simulink model "Clutchless_P2_Parallel_ETE"  (R2017b)
settings: Solver=FixedStepAuto  StartTime=0.0  StopTime=length(Speed)  FixedStep=0.01  MaxStep=0.01  RelTol=1e-3  EnableMultiTasking=on
PostLoadFcn:
  | , if any(exist('dsrtsu_mdlpostloadfcn', 'file') == [2, 3, 6]), try dsrtsu_mdlpostloadfcn('Execute', bdroot); catch fprintf('Error in PostLoadFcn (dsrtsu_mdlpostloadfcn) for model "%s":\n %s\n', bdroot, lasterr); end, end,
undefined symbols (not defined in the file): ABSEnable, Actuators, air, APP1_OOR, APP2_OOR, APP_Mismatch, Brk_Flt, cal, ClutchEngag, Clutchless_HSC_ETE, CS_On_Control, Driver, eng, Engine, EngOverTemp, ENGTRQ_MSMCH_Degraded_CP, ENGTRQ_MSMCH_ErrCritical_CP, ENGTRQ_MSMCH_LimpHome_CP, EngTrqMismatch, env, ess, ESSOverTemp, gb, KeyPos_Flt, KeyPosition, lib_Actuators, lib_Clutchless_HSC_ETE, lib_Driver, lib_EMachine_2017a, lib_Sensors_2017a, LossCAN, Machine, max_vehicle_rad_air_flow, MCUOverTemp, mot, MotDirMismatch, MotOverTemp, MotTrqMismatch, mph2ms, PRNDL_Flt, RegenBrkDisable, RegenFault, Sensors, ShiftLeverPosition, Speed, SW_CS_ON, SW_Engine_ON, t_amb, time, tloop
libraries: simulink x97, Pneumatic_lib x11, nesl_utility x9, EC2_libraries x7, powerlib_meascontrol x2, CalculationGallon x1, lib_Chassis x1, lib_DCDC x1, lib_Differential x1, lib_HVESS x1, fl_lib x1, lib_OBC x1
(part 5 of 9)

== system Clutchless_P2_Parallel_ETE/Clutchless_HSC_ETE/HSC/Camaro Fault Detection/Input Conversions/ECM_Conversions ==
  note: ECM: Input Conversions and Override Switches
      | (Engine and ECM)
  In1 : Inport
  Bus Creator : BusCreator  Inputs=6
  Bus Selector : BusSelector  OutputSignals=from_CAN.fromEBCAN.from_ECM.PlatEngSpdCmdStARC,from_CAN.fromEBCAN.from_ECM.EngSpd,from_CAN.fromEBCAN.from_ECM.EngCltTmp,from_CAN.fromEBCAN.from_ECM.EngRunAtv,from_CAN.fromEBCAN.from_ECM.EngActStdyStTorq
  Conversion  ECMTrqCmd_Nm : DataTypeConversion  OutDataTypeStr=double
  Conversion  EngActStdyStTorq_Nm : DataTypeConversion  OutDataTypeStr=double
  Conversion  EngRunAtv : DataTypeConversion  OutDataTypeStr=boolean
  Conversion  Engine_Speed_rpm : DataTypeConversion  OutDataTypeStr=double
  Conversion  Engine_Temp[DegC] : DataTypeConversion  OutDataTypeStr=double
  Conversion  rollingAliveCnt : DataTypeConversion  OutDataTypeStr=int8
  Memory : Memory
  Override  ECMTrqCmd_Nm : Subsystem
  Override  ECMrollingAliveCnt : Subsystem
  Override  EngActStdyStTorq_Nm : Subsystem
  Override  EngRunAtv : Subsystem
  Override  EngineSpeed_rpm : Subsystem
  Override  Engine_Temp[DegC] : Subsystem
  Out1 : Outport
  wires:
  In1/1 -> Bus Selector/1
  Conversion  rollingAliveCnt/1 -> Override  ECMrollingAliveCnt/1(In1)
  Override  ECMrollingAliveCnt/1(Out1) -> Bus Creator/1  "ECMrollingAliveCnt [123]"
  Bus Creator/1 -> Out1/1  "ECM_Conv"
  Override  ECMTrqCmd_Nm/1(Out1) -> Bus Creator/2  "ECMTrqCmd_Nm"
  Conversion  ECMTrqCmd_Nm/1 -> Override  ECMTrqCmd_Nm/1(In1)
  Bus Selector/2 -> Conversion  Engine_Speed_rpm/1  "<EngSpd>"
  Conversion  Engine_Speed_rpm/1 -> Override  EngineSpeed_rpm/1(In1)
  Override  EngineSpeed_rpm/1(Out1) -> Bus Creator/3  "EngineSpeed_rpm"
  Bus Selector/3 -> Conversion  Engine_Temp[DegC]/1  "<EngCltTmp>"
  Bus Selector/4 -> Conversion  EngRunAtv/1  "<EngRunAtv>"
  Bus Selector/5 -> Conversion  EngActStdyStTorq_Nm/1  "<EngActStdyStTorq>"
  Conversion  Engine_Temp[DegC]/1 -> Override  Engine_Temp[DegC]/1(In1)
  Conversion  EngRunAtv/1 -> Override  EngRunAtv/1(In1)
  Conversion  EngActStdyStTorq_Nm/1 -> Override  EngActStdyStTorq_Nm/1(In1)
  Override  Engine_Temp[DegC]/1(Out1) -> Bus Creator/4  "Engine_Temp[DegC]"
  Override  EngRunAtv/1(Out1) -> Bus Creator/5  "EngRunAtv"
  Override  EngActStdyStTorq_Nm/1(Out1) -> Bus Creator/6  "EngActStdyStTorq_Nm"
  Bus Selector/1 -> Conversion  rollingAliveCnt/1  "<PlatEngSpdCmdStARC>"
  [AxlEngTrqCmd] -> Memory/1
  Memory/1 -> Conversion  ECMTrqCmd_Nm/1

== system Clutchless_P2_Parallel_ETE/Clutchless_HSC_ETE/HSC/Camaro Fault Detection/Input Conversions/TCM_Conversions ==
  note: TCM: Input Conversions and Override Switches
      | (Transmission Control Module)
  In1 : Inport
  Bus Creator : BusCreator  Inputs=4
  Bus Selector : BusSelector  OutputSignals=from_CAN.fromVEH_CAN.from_TCM.TrnsShftLvrPos,from_CAN.fromVEH_CAN.from_TCM.TransEstGear,from_CAN.fromVEH_CAN.from_TCM.TrnsTrqCnvCltCmndMd
  Conversion  LockupCmd : DataTypeConversion  OutDataTypeStr=boolean
  Conversion  LvrPosTrnsShft : DataTypeConversion  OutDataTypeStr=int8
  Conversion  TransEstGear : DataTypeConversion  OutDataTypeStr=int8
  Conversion  rollingAliveCnt : DataTypeConversion  OutDataTypeStr=int8
  Override  LockupCmd : Subsystem
  "Override  LvrPosTrnsShft " : Subsystem
  Override  TransEstGear : Subsystem
  Override  rollingAliveCnt [123] : Subsystem
  TCM_RollinAliveCounter : Subsystem
  Out1 : Outport
  wires:
  Override  LockupCmd/1(Out1) -> Bus Creator/4  "LockupCmd_0_1"
  Conversion  LockupCmd/1 -> Override  LockupCmd/1(In1)
  Bus Selector/3 -> Conversion  LockupCmd/1  "<TrnsTrqCnvCltCmndMd>"
  Override  TransEstGear/1(Out1) -> Bus Creator/3  "TransEstGear"
  Conversion  TransEstGear/1 -> Override  TransEstGear/1(In1)
  Bus Selector/2 -> Conversion  TransEstGear/1  "<TransEstGear>"
  Conversion  LvrPosTrnsShft/1 -> "Override  LvrPosTrnsShft "/1(In1)
  "Override  LvrPosTrnsShft "/1(Out1) -> Bus Creator/2  "LvrPosTrnsShft"
  Bus Selector/1 -> Conversion  LvrPosTrnsShft/1  "<TrnsShftLvrPos>"
  Bus Creator/1 -> Out1/1  "TCM_Conv"
  Override  rollingAliveCnt [123]/1(Out1) -> Bus Creator/1  "TCMrollingAliveCnt [123]"
  Conversion  rollingAliveCnt/1 -> Override  rollingAliveCnt [123]/1(In1)
  In1/1 -> Bus Selector/1
  TCM_RollinAliveCounter/1(Out1) -> Conversion  rollingAliveCnt/1

== system Clutchless_P2_Parallel_ETE/Clutchless_HSC_ETE/HSC/Camaro Fault Detection/Signal Diagnostic/Driver Signal Diagnostic ==
  note: Driver Controls : Signal Diagnostic
  Sensors1 : Inport
  APP_Crosscheck : Subsystem
  AccPedalValidity : Stateflow chart  TreatAsAtomicUnit=on
  AccPedalValidity1 : Stateflow chart  TreatAsAtomicUnit=on
  BPP_faild_ovrd : Constant  Value=0  OutDataTypeStr=boolean
  BrakeFailureDetection : Subsystem
  Bus Creator : BusCreator  Inputs=7
  Bus Selector : BusSelector  OutputSignals=DriverControls_Conv.APP1 [%],DriverControls_Conv.APP2[%],DriverControls_Conv.BPP [%],DriverControls_Conv.V [mph],DriverControls_Conv.keyPos [0_3],DriverControls_Conv.PRNDL
  ClearAPP1fault : Constant  Value=0
  ClearAPP2fault : Constant  Value=0
  Constant2 : Constant  Value=0
  Constant3 : Constant  OutDataTypeStr=boolean
  Conversion  APP1 (%)1 : DataTypeConversion  OutDataTypeStr=boolean
  Conversion  APP1 (%)2 : DataTypeConversion
  Conversion  APP1 (%)3 : DataTypeConversion
  Drv_APP1_valid_ovrd : Constant  Value=0  OutDataTypeStr=boolean
  Drv_APP2_valid_ovrd : Constant  Value=0  OutDataTypeStr=boolean
  Interval Test : simulink/Logic and Bit Operations/Interval Test  IntervalClosedRight=on  uplimit=100  IntervalClosedLeft=on  lowlimit=0  OutDataTypeStr=boolean
  Interval Test1 : simulink/Logic and Bit Operations/Interval Test  IntervalClosedRight=on  uplimit=3  IntervalClosedLeft=on  lowlimit=0  OutDataTypeStr=boolean
  Interval Test2 : simulink/Logic and Bit Operations/Interval Test  IntervalClosedRight=on  uplimit=4  IntervalClosedLeft=on  lowlimit=0  OutDataTypeStr=boolean
  Latch : Subsystem
  Latch1 : Subsystem
  Logical Operator1 : Logic  AllPortsSameDT=off  OutDataTypeStr=boolean
  Logical Operator5 : Logic  Operator=OR  AllPortsSameDT=off  OutDataTypeStr=boolean
  Logical Operator6 : Logic  Operator=OR  AllPortsSameDT=off  OutDataTypeStr=boolean
  Pulse Generator : DiscretePulseGenerator  PulseType=Time based  Period=0.1  PulseWidth=10
  Scope : Scope
  Driver_SigDiag : Outport
  wires:
  Sensors1/1 -> Bus Selector/1
  Bus Selector/1 -> AccPedalValidity/2(signalValue), APP_Crosscheck/1(In1)  "<APP1 [%]>"
  Bus Selector/2 -> AccPedalValidity1/2(signalValue), APP_Crosscheck/2(In2)  "<APP2[%]>"
  ClearAPP1fault/1 -> AccPedalValidity/1(clearFaults)
  ClearAPP2fault/1 -> AccPedalValidity1/1(clearFaults)
  Bus Selector/3 -> Interval Test/1, BrakeFailureDetection/1(BPP)  "<BPP [%]>"
  Bus Selector/5 -> Interval Test1/1  "<keyPos [0_3]>"
  Logical Operator6/1 -> Bus Creator/1  "Drv_APP1_[%]_SigValid"
  Interval Test/1 -> Bus Creator/4  "Drv_BPP_[%]_SigValid"
  Logical Operator5/1 -> Bus Creator/2  "Drv_APP2_[%]_SigValid"
  Bus Creator/1 -> Driver_SigDiag/1  "Driver_SignalDiag"
  Bus Selector/6 -> Interval Test2/1  "<PRNDL>"
  Constant3/1 -> Latch/2(In2)
  APP_Crosscheck/1(Out1) -> Latch/1(In1)  "Drv_APP_Agree"
  Bus Selector/4 -> BrakeFailureDetection/2(VehSpeed)  "<V [mph]>"
  Constant2/1 -> Conversion  APP1 (%)1/1
  Conversion  APP1 (%)1/1 -> Latch1/2(In2)
  BrakeFailureDetection/1(DecelFail) -> Latch1/1(In1)  "Brake_Failed"
  Interval Test2/1 -> Bus Creator/7  "Drv_PRNDL_SigValid"
  Drv_APP2_valid_ovrd/1 -> Logical Operator5/1
  AccPedalValidity1/1(signalValid) -> Logical Operator5/2  "Drv_APP2_[%]_SigValid"
  Drv_APP1_valid_ovrd/1 -> Logical Operator6/1
  AccPedalValidity/1(signalValid) -> Logical Operator6/2  "Drv_APP1_[%]_SigValid"
  Conversion  APP1 (%)3/1 -> Bus Creator/3  "Drv_APP_Agree"
  Conversion  APP1 (%)2/1 -> Bus Creator/5  "Brake_Failed"
  Interval Test1/1 -> Bus Creator/6  "Drv_KeyPos_[0 3]_SigValid"
  Latch/1(Drv_APP_Agree) -> Conversion  APP1 (%)3/1  "Drv_APP_Agree"
  Logical Operator1/1 -> Conversion  APP1 (%)2/1  "Brake_Failed"
  Latch1/1(Out1) -> Logical Operator1/2  "Brake_Failed"
  BPP_faild_ovrd/1 -> Logical Operator1/1
  Pulse Generator/1 -> BrakeFailureDetection/Trigger, Scope/1

== system Clutchless_P2_Parallel_ETE/Clutchless_HSC_ETE/HSC/Camaro Fault Detection/Signal Diagnostic/ESS Signal Diagnostic ==
  note: max charge current: 180A
      | Max discharge current: 315A;
  note: Error: contactors welded,Contactors don't close when commanded
  note: Temperature Range check :
      | 0 = below normal operation (<-28)
      | 1 = low range (<0 - >-28)
      | 2 = normal range (0 -30 C)
      | 3= high range (>30)
      | 4= above max value allowed (>55)
  note: SOC Range check definition :
      | 0 = below normal operation (<0.15)
      | 1 = low range ([0.15 0.30])
      | 2 = normal range (0.3)
      | 3= SOC high/full (>0.95)
  note: 1) Rolling alive detection : is the component on and transmitting?
      | 2) Probably move the voltage check to component diagnostic (no signal from Bosch to check the contactors status)
      | 3) Is  the T signal within an acceptable range?
  note: BMS : Signal Diagnostic
  Sensors1 : Inport
  Bus Creator : BusCreator  Inputs=14
  Bus Selector : BusSelector  OutputSignals=BMS_Conv.BMSrollingAliveCnt [123],BMS_Conv.hvBattVolt_V,BMS_Conv.hvBusVolt_V,BMS_Conv.Fehler_HS_offen,BMS_Conv.MO_BMS_Sollmodus [0-5],BMS_Conv.Fehler_HS_verschweisst,BMS_Conv.essTemp_C,BMS_Conv.essSOC_0_1,BMS_Conv.essCur_A,BMS_Conv.BMS_gdf
  Contactors status check : Subsystem
  ESS SOC Validity Check : Subsystem
  ESS Temp Validity Check : Subsystem
  Interval Test : simulink/Logic and Bit Operations/Interval Test  IntervalClosedRight=on  uplimit=180  IntervalClosedLeft=on  lowlimit=-315  OutDataTypeStr=boolean
  Interval Test1 : simulink/Logic and Bit Operations/Interval Test  IntervalClosedRight=on  uplimit=7  IntervalClosedLeft=on  lowlimit=0  OutDataTypeStr=boolean
  Interval Test2 : simulink/Logic and Bit Operations/Interval Test  IntervalClosedRight=on  uplimit=430  IntervalClosedLeft=on  lowlimit=291  OutDataTypeStr=boolean
  Logical Operator : Logic  Operator=OR  AllPortsSameDT=off  OutDataTypeStr=boolean
  Max charging voltage fault detect : Subsystem
  Override_ BMS_RACvalid1 : Constant  Value=0
  Rolling Alive Counter Detection : Subsystem
  Validity Check : Subsystem
  ESS_SigDiag : Outport
  wires:
  Sensors1/1 -> Bus Selector/1
  Bus Selector/1 -> Rolling Alive Counter Detection/1(In1)  "<BMSrollingAliveCnt [123]>"
  Logical Operator/1 -> Bus Creator/1  "BMS_RollingAliveActive_SigValid"
  Bus Selector/2 -> Interval Test2/1, [BattVolt]  "<hvBattVolt_V>"
  Bus Creator/1 -> ESS_SigDiag/1  "ESS_SignalDiag"
  Bus Selector/9 -> Interval Test/1  "<essCur_A>"
  Interval Test/1 -> Bus Creator/12  "essCur_A_SigValid"
  Bus Selector/10 -> Bus Creator/14, Validity Check/1(In1)  "<BMS_gdf>"
  Validity Check/1(Out1) -> Bus Creator/13  "BMSgdf_SigValid"
  Bus Selector/8 -> ESS SOC Validity Check/1(In1)  "<essSOC_0_1>"
  ESS SOC Validity Check/1(Out1) -> Bus Creator/10
  ESS SOC Validity Check/2(Out2) -> Bus Creator/11
  Bus Selector/7 -> ESS Temp Validity Check/1(In1)  "<essTemp_C>"
  ESS Temp Validity Check/1(Out1) -> Bus Creator/8
  ESS Temp Validity Check/2(Out2) -> Bus Creator/9
  Bus Selector/3 -> Contactors status check/2(In2), [BusVolt]  "<hvBusVolt_V>"
  Bus Selector/4 -> Contactors status check/3(In3)  "<Fehler_HS_offen>"
  Contactors status check/1(Out1) -> Bus Creator/4  "BMS_contactorsFailed_Detected"
  Bus Selector/6 -> Bus Creator/7  "<Fehler_HS_verschweisst>"
  Bus Selector/5 -> Interval Test1/1  "<MO_BMS_Sollmodus [0-5]>"
  Interval Test1/1 -> Bus Creator/6  "Contatctors_Status_Validity"
  Interval Test2/1 -> Bus Creator/2  "OverVolt_Detected"
  [BattVolt] -> Contactors status check/1(In1)
  [BusVolt] -> Max charging voltage fault detect/1(In1)
  Max charging voltage fault detect/1(Out1) -> Bus Creator/5  "ChargVoltFlt"
  [BusVolt] -> Bus Creator/3  "hvBusVolt_V"
  Rolling Alive Counter Detection/1(Out1) -> Logical Operator/2  "BMS_RollingAliveActive_SigValid"
  Override_ BMS_RACvalid1/1 -> Logical Operator/1

== system Clutchless_P2_Parallel_ETE/Clutchless_HSC_ETE/HSC/Camaro Fault Detection/Signal Diagnostic/Engine Signal Diagnostic ==
  note: ECM : Signal Diagnostic
  note: Engine_Temp:
      | Normal range: <100
      | above max:>120
      | Limited range: 100-120
  Sensors1 : Inport
  Bus Creator : BusCreator  Inputs=9
  Bus Selector : BusSelector  OutputSignals=ECM_Conv.ECMrollingAliveCnt [123],ECM_Conv.ECMTrqCmd_Nm,ECM_Conv.EngActStdyStTorq_Nm,ECM_Conv.EngineSpeed_rpm,ECM_Conv.Engine_Temp[DegC],ECM_Conv.EngRunAtv
  Constant1 : Constant
  EngTempValidity_Check : Subsystem
  Engine_Temp[DegC] : Stateflow chart  TreatAsAtomicUnit=on
  Interval Test : simulink/Logic and Bit Operations/Interval Test  IntervalClosedRight=on  uplimit=233  IntervalClosedLeft=on  lowlimit=0  OutDataTypeStr=boolean
  Interval Test1 : simulink/Logic and Bit Operations/Interval Test  IntervalClosedRight=on  uplimit=6500  IntervalClosedLeft=on  lowlimit=0  OutDataTypeStr=boolean
  Interval Test2 : simulink/Logic and Bit Operations/Interval Test  IntervalClosedRight=on  uplimit=233  IntervalClosedLeft=on  lowlimit=0  OutDataTypeStr=boolean
  Interval Test3 : simulink/Logic and Bit Operations/Interval Test  IntervalClosedRight=on  uplimit=1  IntervalClosedLeft=on  lowlimit=0  OutDataTypeStr=boolean
  Rolling Alive Counter Detection1 : Subsystem
  Engine_SigDiag : Outport
  wires:
  Sensors1/1 -> Bus Selector/1
  Bus Selector/1 -> Rolling Alive Counter Detection1/1(In1)  "<ECMrollingAliveCnt [123]>"
  Rolling Alive Counter Detection1/1(Out1) -> Bus Creator/1  "ECMRollingAliveActive"
  Bus Selector/2 -> Bus Creator/2, Interval Test/1  "<ECMTrqCmd_Nm>"
  Interval Test/1 -> Bus Creator/3  "engTrqCmdRecvd_SigValid"
  Bus Creator/1 -> Engine_SigDiag/1  "Engine_SignalDiag"
  Bus Selector/4 -> Interval Test1/1  "<EngineSpeed_rpm>"
  Interval Test1/1 -> Bus Creator/6  "Engine_Speed_rpm_SigValid"
  Bus Selector/3 -> Bus Creator/5, Interval Test2/1  "<EngActStdyStTorq_Nm>"
  Interval Test2/1 -> Bus Creator/4  "EngActStdyStTorq_SigValid"
  Bus Selector/5 -> Engine_Temp[DegC]/2(Engine_Temp_DegC)  "<Engine_Temp[DegC]>"
  Bus Selector/6 -> Interval Test3/1  "<EngRunAtv>"
  Interval Test3/1 -> Bus Creator/9  "EngRunAtValid"
  Constant1/1 -> Engine_Temp[DegC]/1(clearFaults)
  Engine_Temp[DegC]/1(EngTempRange) -> EngTempValidity_Check/1(In1), Bus Creator/8  "Eng_TempRange[123]"
  EngTempValidity_Check/1(Out1) -> Bus Creator/7  "Eng_TempValid"

== system Clutchless_P2_Parallel_ETE/Clutchless_HSC_ETE/HSC/Camaro Fault Detection/Signal Diagnostic/Subsystem1 ==
  note: Signal Valid Setting Rule
      | xxx_yyy_[z]_SigValid could be 0 or 1
      | 0: signal invalid
      | 1: signal vaild
  note: Signal Naming Rule
      | Example: xxx_yyy_[z]_SigValid
      | xxx: source of the signal (Drv, Clu, BCM, ECM, TCM, BMS and MCU)
      | yyy: description of the signal
      | z: unit of the signal (V, A, Nm, m/s, %, 01, 0123, etc.)

== system Clutchless_P2_Parallel_ETE/Clutchless_HSC_ETE/HSC/Camaro Fault Detection/Signal Diagnostic/Transmission Signal Diagnostic ==
  note: TCM : Signal Diagnostic
  note: TransEstGear
      | 0 : Not Supported
      | 1 : First Gear
      | 2 : Second Gear
      | 3 : Third Gear
      | 4 : Fourth Gear
      | 5 : Fifth Gear
      | 6 : Sixth Gear
      | 7 : Seventh Gear
      | 8 : Eight Gear
      | 10: EVT Mode 1
      | 11: EVT Mode 2
      | 12: CVT Forward Gear
      | 13: Neutral Gear
      | 14: Reverse Gear
      | 15: Park Gear
  note: Lever Position:
      | 1 P
      | 2 R
      | 3 N
      | 4 D
      | 0: L
  Sensors1 : Inport
  Bus Creator : BusCreator  Inputs=5
  Bus Selector : BusSelector  OutputSignals=TCM_Conv.TCMrollingAliveCnt [123],TCM_Conv.LvrPosTrnsShft,TCM_Conv.TransEstGear,DriverControls_Conv.V [mph],TCM_Conv.LockupCmd_0_1
  Interval Test : simulink/Logic and Bit Operations/Interval Test  IntervalClosedRight=on  uplimit=4  IntervalClosedLeft=on  lowlimit=0  OutDataTypeStr=boolean
  Interval Test1 : simulink/Logic and Bit Operations/Interval Test  IntervalClosedRight=on  uplimit=15  IntervalClosedLeft=on  lowlimit=0  OutDataTypeStr=boolean
  Interval Test2 : simulink/Logic and Bit Operations/Interval Test  IntervalClosedRight=on  uplimit=1  IntervalClosedLeft=on  lowlimit=0  OutDataTypeStr=boolean
  Rolling Alive Counter Detection : Subsystem
  Vehicle Direction Fault Detection : Subsystem
  Out2 : Outport
  wires:
  Bus Selector/4 -> Vehicle Direction Fault Detection/2(Speed)  "<V [mph]>"
  Sensors1/1 -> Bus Selector/1
  Bus Selector/1 -> Rolling Alive Counter Detection/1(In1)  "<TCMrollingAliveCnt [123]>"
  Rolling Alive Counter Detection/1(Out1) -> Bus Creator/1  "TCMRollingAliveActive_SigValid"
  Bus Creator/1 -> Out2/1
  Bus Selector/2 -> Vehicle Direction Fault Detection/1(LvrPosTrnsShft), Interval Test/1  "<LvrPosTrnsShft>"
  Bus Selector/3 -> Interval Test1/1  "<TransEstGear>"
  Bus Selector/5 -> Interval Test2/1  "<LockupCmd_0_1>"
  Interval Test/1 -> Bus Creator/2  "LvrPosTrnsShft_SigValid"
  Interval Test1/1 -> Bus Creator/3  "TransEstGear_SigValid"
  Interval Test2/1 -> Bus Creator/5  "LockupCmd_SigValid"
  Vehicle Direction Fault Detection/1(Out1) -> Bus Creator/4  "VehDirFault"

== system Clutchless_P2_Parallel_ETE/Clutchless_HSC_ETE/HSC/Driver_Requests/APP_BPP to DrvIntndAxlTrq2/Post Driver Intnded Axle Torque ==
  note: //*mode==1 (CD Mode)
      | mode==2 (CS Mode - Engine Drive)
      | mode==3 (CS Mode-Motor Drive) pass MotTrq
      | mode==4 (Sports Mode) pass Mot Trq+Eng Trq
      | mode==5 (Engine only mode)*//
  APP : Inport
  BPP : Inport  Port=2
  VehicleSpeed : Inport  Port=3
  TransGearRatio : Inport  Port=4
  Mode : Inport  Port=5
  Motor_Speed : Inport  Port=6
  APP1 : InportShadow
  Abs : Abs
  Add : Sum
  Brake Command : Subsystem
  Bus Creator1 : BusCreator  Inputs=1
  Bus Creator3 : BusCreator  Inputs=3
  Driver Intended Axle Torque : Subsystem
  Switch : Switch  Threshold=cal.Regen.MinMotSpd
  rad/s to RPM2 : Gain  Gain=30/pi
  IntndAxlTrq : Outport
  BrkIntndAxlTrq : Outport  Port=2
  tag scope: DrvIntdAxleTrq=global
  wires:
  rad/s to RPM2/1 -> Abs/1
  [DrvIntdAxleTrq] -> Switch/3
  APP1/1 -> Driver Intended Axle Torque/1(APP)
  [DrvIntdAxleTrq] -> Bus Creator3/2
  Bus Creator3/1 -> IntndAxlTrq/1  "IntndAxlTrq"
  Switch/1 -> Bus Creator3/1  "FullDrvIntndAxlTrq"
  Add/1 -> Switch/1  "FullDrvIntndAxlTrq"
  Abs/1 -> Switch/2
  Motor_Speed/1 -> rad/s to RPM2/1
  Bus Creator1/1 -> BrkIntndAxlTrq/1
  Brake Command/1(BrkAxlTrq) -> Bus Creator3/3, Bus Creator1/1, Add/2  "BrkIntndAxlTrq"
  TransGearRatio/1 -> Driver Intended Axle Torque/3(TransGearRatio)
  Mode/1 -> Driver Intended Axle Torque/2(Mode)
  VehicleSpeed/1 -> Brake Command/3(VehicleSpeed)
  BPP/1 -> Brake Command/2(BPP)
  Driver Intended Axle Torque/1(Out1) -> [DrvIntdAxleTrq], Add/1  "DrvIntndAxlTrq"
  APP/1 -> Brake Command/1(APP)

== system Clutchless_P2_Parallel_ETE/Clutchless_HSC_ETE/HSC/Powertrain Manager/HV Manager1/Axiomatic_Output_Manager ==
  Sensors : Inport
  HV_Bus_Status : Inport  Port=2
  BrkPumpOffVal : Constant  Value=0
  BrkPumpOnVal : Constant
  Bus Creator : BusCreator  Inputs=4
  Bus Selector : BusSelector  OutputSignals=GFD_Light
  Bus Selector1 : BusSelector  OutputSignals=from_CAN.fromEBCAN.from_ECM.EngRunAtv
  Bus Selector2 : BusSelector  OutputSignals=from_CAN.fromVEH_CAN.from_BCM.SysPwrMd
  Bus Selector5 : BusSelector  OutputSignals=from_CAN.fromHV_CAN.from_OBC.NLG5_ST.NLG5_S_CP_DT
  Compare To Constant : simulink/Logic and Bit Operations/Compare To Constant  relop===  const=2  OutDataTypeStr=boolean
  Compare To Constant1 : simulink/Logic and Bit Operations/Compare To Constant  relop===  const=1  OutDataTypeStr=boolean
  Data Type Conversion : DataTypeConversion
  Data Type Conversion1 : DataTypeConversion
  Logical Operator : Logic  AllPortsSameDT=off  OutDataTypeStr=boolean
  Logical Operator1 : Logic  Operator=NOT  AllPortsSameDT=off  OutDataTypeStr=boolean
  Sensors1 : InportShadow
  Sensors2 : InportShadow
  Switch : Switch  Criteria=u2 ~= 0
  Axiomatic_CAN : Outport
  wires:
  Data Type Conversion1/1 -> Bus Creator/4  "Brake_Pump_Switch"
  Switch/1 -> Data Type Conversion1/1
  BrkPumpOffVal/1 -> Switch/3
  BrkPumpOnVal/1 -> Switch/1
  Compare To Constant/1 -> Switch/2
  Bus Selector2/1 -> Compare To Constant/1  "<SysPwrMd>"
  Sensors2/1 -> Bus Selector2/1
  Sensors1/1 -> Bus Selector5/1
  Bus Selector1/1 -> Compare To Constant1/1  "<EngRunAtv>"
  Bus Selector5/1 -> Logical Operator1/1  "<NLG5_S_CP_DT>"
  Logical Operator1/1 -> Logical Operator/1
  Compare To Constant1/1 -> Logical Operator/2
  HV_Bus_Status/1 -> Bus Selector/1
  Bus Creator/1 -> Axiomatic_CAN/1  "Axiomatic_CAN"
  Bus Selector/1 -> Bus Creator/1  "<GFD_Light>"
  Data Type Conversion/1 -> Bus Creator/2  "HV_Chg_Light"
  Logical Operator/1 -> Bus Creator/3  "Veh_Ready_Light"
  Sensors/1 -> Bus Selector1/1
  [HV_Charge_Indicator] -> Data Type Conversion/1

== system Clutchless_P2_Parallel_ETE/Clutchless_HSC_ETE/HSC/Powertrain Manager/HV Manager1/BMS_Manager ==
  Sensors : Inport
  Controls : Inport  Port=2
  In1 : Inport  Port=3
  Bus Creator : BusCreator  Inputs=3
  Bus Creator1 : BusCreator  Inputs=8
  Bus Creator2 : BusCreator  Inputs=2
  Bus Creator3 : BusCreator  Inputs=6
  Bus Creator4 : BusCreator  Inputs=5
  Bus Selector : BusSelector  OutputSignals=closeMaincReq
  Bus Selector1 : BusSelector  OutputSignals=from_CAN.fromHV_CAN.from_BMSHybrid.BMS_HYB_02.BMS_Fehler_HS_offen,from_CAN.fromHV_CAN.from_BMSHybrid.BMS_HYB_02.BMS_Fehler_Pilot,from_CAN.fromHV_CAN.from_BMSHybrid.BMS_HYB_02.BMS_Init_abgeschlossen,from_CAN.fromHV_CAN.from_BMSHybrid.BMS_HYB_02.BMS_IstModus,from_CAN.fromHV_CAN.from_BMSHybrid.BMS_HYB_02.BMS_IstSpannung,from_CAN.fromHV_CAN.from_BMSHybrid.BMS_HYB_02.BMS_IstStrom,from_CAN.fromHV_CAN.from_BMSHybrid.BMS_HYB_02.BMS_SleepInd
  Bus Selector2 : BusSelector  OutputSignals=from_CAN.fromEBCAN.from_BMSAntrieb.NMH_BMS.NMH_BMS_Car_WakeUp,from_CAN.fromEBCAN.from_BMSAntrieb.NMH_BMS.NMH_BMS_Normal_Mode_1,from_CAN.fromEBCAN.from_BMSAntrieb.NMH_BMS.NMH_BMS_Normal_Mode_2,from_CAN.fromEBCAN.from_BMSAntrieb.NMH_BMS.NMH_BMS_Start_1,from_CAN.fromEBCAN.from_BMSAntrieb.NMH_BMS.NMH_BMS_Start_2,from_CAN.fromVEH_CAN.from_BCM.SysPwrMd,from_CAN.fromEBCAN.from_ECM.EngRunAtv
  Bus Selector3 : BusSelector  OutputSignals=from_CAN.fromHV_CAN.from_BMSHybrid.BMS_Spannung_ZwKr
  Bus Selector4 : BusSelector  OutputSignals=HV_req
  Bus Selector5 : BusSelector  OutputSignals=from_CAN.fromHV_CAN.from_OBC.NLG5_ST.NLG5_S_CP_DT
  Bus Selector6 : BusSelector  OutputSignals=from_CAN.fromHV_CAN.from_MCU.INV_VCU_01.INV_State
  Bus Selector7 : BusSelector  OutputSignals=MCU_State
  Bus Selector8 : BusSelector  OutputSignals=from_CAN.fromHV_CAN.from_BMSHybrid.BMS_SOC
  Controls1 : InportShadow  Port=2
  Data Type Conversion{,1,6..8} (5 alike) : DataTypeConversion  OutDataTypeStr=boolean
  ESS_Manager : Stateflow chart  TreatAsAtomicUnit=on
  Edge Detector : powerlib_meascontrol/Logic/Edge Detector  model=Either  ic=0  Ts=0
      settings: SourceProductName=Simscape Power Systems  SourceProductBaseCode=PS
  Fault Latch : Subsystem
  ISO_Hybrid_01_Req : Subsystem
  Isolation Fault Calculation : Subsystem
  Memory : Memory
  Memory1 : Memory
  BMS CAN : Outport
  HV_BUS_Status : Outport  Port=2
  BMS Digital : Outport  Port=3
  wires:
  Memory1/1 -> ESS_Manager/22(MCU_State)
  Memory/1 -> Data Type Conversion7/1
  Bus Selector7/1 -> Memory1/1  "<MCU_State>"
  In1/1 -> Bus Selector7/1
  Sensors/1 -> Bus Selector1/1, Bus Selector5/1, Isolation Fault Calculation/1(Sensors1), Bus Selector3/1, Bus Selector2/1, Bus Selector6/1, Bus Selector8/1
  Bus Selector8/1 -> ESS_Manager/21(SoC)  "<BMS_SOC>"
  Bus Selector6/1 -> ESS_Manager/20(INV_State)  "<INV_State>"
  ESS_Manager/22(GFD_Light) -> Bus Creator3/6  "GFD_Light"
  Data Type Conversion/1 -> ESS_Manager/2(plugged)
  Bus Selector1/6 -> ESS_Manager/8(BMS_IstStrom)  "<BMS_IstStrom>"
  Bus Selector1/7 -> ESS_Manager/9(BMS_SleepInd)  "<BMS_SleepInd>"
  Bus Selector2/4 -> ESS_Manager/15(NMH_BMS_Start_1)  "<NMH_BMS_Start_1>"
  Bus Selector2/5 -> ESS_Manager/16(NMH_BMS_Start_2)  "<NMH_BMS_Start_2>"
  Bus Selector2/7 -> ESS_Manager/18(EngRunAtv)  "<EngRunAtv>"
  Edge Detector/1 -> ESS_Manager/17(KeyPos)
  Bus Selector2/6 -> Edge Detector/1  "<SysPwrMd>"
  Bus Selector4/1 -> ESS_Manager/10(HV_req)  "<HV_req>"
  Bus Creator2/1 -> Bus Creator/3  "MSG_HYB_01"
  Fault Latch/1(IsoFaultLatched) -> ESS_Manager/1(ISOfault)
  Isolation Fault Calculation/1(IsoFault) -> Fault Latch/1(IsoFault)
  Bus Selector1/1 -> ESS_Manager/3(BMS_Fehler_HS_offen)  "<BMS_Fehler_HS_offen>"
  Bus Selector1/2 -> ESS_Manager/4(BMS_Fehler_Pilot)  "<BMS_Fehler_Pilot>"
  Bus Selector1/3 -> ESS_Manager/5(BMS_Init_abgeschlossen)  "<BMS_Init_abgeschlossen>"
  Bus Selector1/4 -> ESS_Manager/6(BMS_IstModus)  "<BMS_IstModus>"
  Bus Selector1/5 -> ESS_Manager/7(BMS_IstSpannung)  "<BMS_IstSpannung>"
  Bus Selector2/1 -> ESS_Manager/12(NMH_BMS_Car_WakeUp)  "<NMH_BMS_Car_WakeUp>"
  Bus Selector2/2 -> ESS_Manager/13(NMH_Normal_Mode_1)  "<NMH_BMS_Normal_Mode_1>"
  Bus Selector2/3 -> ESS_Manager/14(NMH_BMS_Normal_Mode_2)  "<NMH_BMS_Normal_Mode_2>"
  Bus Selector3/1 -> ESS_Manager/11(BMS_Spannung_ZwKr)  "<BMS_Spannung_ZwKr>"
  Bus Selector5/1 -> Data Type Conversion/1  "<NLG5_S_CP_DT>"
  ESS_Manager/1(Diag_Rq_Fktnl_Data_OBD_byte_0) -> Bus Creator1/1
  ESS_Manager/2(Diag_Rq_Fktnl_Data_OBD_byte_1) -> Bus Creator1/2
  ESS_Manager/3(Diag_Rq_Fktnl_Data_OBD_byte_2) -> Bus Creator1/3
  ESS_Manager/4(Diag_Rq_Fktnl_Data_OBD_byte_3) -> Bus Creator1/4
  ESS_Manager/5(Diag_Rq_Fktnl_Data_OBD_byte_4) -> Bus Creator1/5
  ESS_Manager/6(Diag_Rq_Fktnl_Data_OBD_byte_5) -> Bus Creator1/6
  ESS_Manager/7(Diag_Rq_Fktnl_Data_OBD_byte_6) -> Bus Creator1/7
  ESS_Manager/8(Diag_Rq_Fktnl_Data_OBD_byte_7) -> Bus Creator1/8
  ESS_Manager/10(MO_SleepAckn) -> Bus Creator2/1
  ESS_Manager/12(T_15) -> Bus Creator4/1
  Data Type Conversion6/1 -> Bus Creator3/3  "ReadyToDrive"
  Data Type Conversion7/1 -> Bus Creator3/4  "ReadyToCharge"
  Data Type Conversion8/1 -> Bus Creator3/1  "HV Discharge"
  Bus Creator1/1 -> Bus Creator/1  "ISO_Funktionaler_Req_All"
  ESS_Manager/17(HVDischarge) -> Data Type Conversion8/1
  ESS_Manager/19(ReadyToDrive) -> Data Type Conversion6/1
  ESS_Manager/20(ReadyToCharge) -> Memory/1
  ESS_Manager/21(Shutdown_Complete) -> Bus Creator3/5
  ESS_Manager/13(T_30) -> Bus Creator4/2
  ESS_Manager/16(chga_wake) -> Data Type Conversion1/1
  ESS_Manager/14(T_30C) -> Bus Creator4/3
  ESS_Manager/15(veh_wake) -> Bus Creator4/4
  ESS_Manager/18(HV_State) -> Bus Creator3/2
  Bus Creator3/1 -> HV_BUS_Status/1  "HV_BUS_Status"
  Controls/1 -> Bus Selector/1
  Bus Selector/1 -> ESS_Manager/19(closeMaincReq)  "<closeMaincReq>"
  Controls1/1 -> Bus Selector4/1
  Bus Creator/1 -> BMS CAN/1  "BMS_CAN"
  Bus Creator4/1 -> BMS Digital/1  "BMS_Digital"
  Data Type Conversion1/1 -> Bus Creator4/5  "chg_wake"
  ESS_Manager/11(MO_BMS_Sollmodus) -> Bus Creator2/2
  ESS_Manager/9(ISO_Hybrid_01_Req) -> ISO_Hybrid_01_Req/1(In1)
  ISO_Hybrid_01_Req/1(Out1) -> Bus Creator/2

== system Clutchless_P2_Parallel_ETE/Clutchless_HSC_ETE/HSC/Powertrain Manager/HV Manager1/DCDC Manager ==
  BMSInput : Inport
  In1 : Inport  Port=2
  In2 : Inport  Port=3
  Bus Creator : BusCreator  Inputs=6
  Bus Selector : BusSelector  OutputSignals=from_CAN.fromHV_CAN.from_MCU.INV_VCU_01.INV_State
  Bus Selector1 : BusSelector  OutputSignals=from_CAN.fromHV_CAN.from_BMSHybrid.BMS_HYB_02.BMS_IstModus
  Bus Selector2 : BusSelector  OutputSignals=EngOnReq,powerMode,mode
  Bus Selector3 : BusSelector  OutputSignals=HV_req
  Bus Selector4 : BusSelector  OutputSignals=from_CAN.fromVEH_CAN.from_BCM.SysPwrMd
  Chart : Stateflow chart  RequirementInfo={} %GIDa_3890bf8e_4224_46d0_98ba_a4f91d8dccc7  TreatAsAtomicUnit=on
  Contactors status check : Subsystem
  Override_Current : Subsystem
  Override_CurrentLV : Subsystem
  Override_Voltage : Subsystem
  Override_VoltageLV : Subsystem
  Override_mode : Subsystem
  Out1 : Outport
  wires:
  Contactors status check/1(Out1) -> Chart/8(ContactorsFailed)  "ContactorsFailed"
  Bus Selector4/1 -> Chart/7(keypos)  "<SysPwrMd>"
  Override_CurrentLV/1(Out1) -> Bus Creator/5  "CurrentLV"
  Override_VoltageLV/1(Out1) -> Bus Creator/4  "VoltageLV"
  Override_Current/1(Out1) -> Bus Creator/3  "CurrentHV"
  Override_Voltage/1(Out1) -> Bus Creator/2  "VoltageHV"
  Override_mode/1(Out1) -> Bus Creator/1  "DC_mode"
  Chart/1(DCmode) -> Override_mode/1(In1)  "DC_mode"
  Bus Selector2/3 -> Chart/6(mode)  "<mode>"
  Bus Selector3/1 -> Chart/2(CloseMainC)  "<HV_req>"
  In2/1 -> Bus Selector3/1
  Bus Selector2/1 -> Chart/4(EngOnReq)  "<EngOnReq>"
  Bus Selector1/1 -> Chart/1(BMS_IstModus)  "<BMS_IstModus>"
  Bus Selector2/2 -> Chart/5(powerMode)  "<powerMode>"
  In1/1 -> Bus Selector2/1
  Chart/6(DCDC_State) -> Bus Creator/6  "DCDC_State"
  Bus Creator/1 -> Out1/1  "DCDC_Out"
  Chart/2(VoltageHV) -> Override_Voltage/1(In1)  "VoltageHV"
  Chart/3(CurrentHV) -> Override_Current/1(In1)  "CurrentHV"
  Chart/4(VoltageLV) -> Override_VoltageLV/1(In1)  "VoltageLV"
  Chart/5(CurrentLV) -> Override_CurrentLV/1(In1)  "CurrentLV"
  Bus Selector/1 -> Chart/3(INV_state)  "<INV_State>"
  BMSInput/1 -> Bus Selector1/1, Bus Selector/1, Bus Selector4/1, Contactors status check/1(In1)

== system Clutchless_P2_Parallel_ETE/Clutchless_HSC_ETE/HSC/Powertrain Manager/HV Manager1/Inverter Manager ==
  HV_Bus_Status : Inport
  Sensors : Inport  Port=2
  Control : Inport  Port=3
  Bus Creator2 : BusCreator  Inputs=1
  Bus Creator3 : BusCreator  Inputs=2
  Bus Creator4 : BusCreator  Inputs=1
  Bus Selector : BusSelector  OutputSignals=ReadyToDrive,ReadyToCharge,HV_State
  Bus Selector1 : BusSelector  OutputSignals=EnableInverter
  Bus Selector3 : BusSelector  OutputSignals=from_CAN.fromHV_CAN.from_MCU.INV_VCU_01.MessageCounter_200,from_CAN.fromVEH_CAN.from_BCM.SysPwrMd,from_CAN.fromHV_CAN.from_BMSHybrid.BMS_Spannung_ZwKr,from_CAN.fromHV_CAN.from_MCU.INV_VCU_01.INV_State,from_CAN.fromHV_CAN.from_MCU.INV_VCU_01.INV_CurrentHV
  Data Type Conversion : DataTypeConversion  OutDataTypeStr=boolean
  Data Type Conversion1 : DataTypeConversion  OutDataTypeStr=boolean
  Data Type Conversion2 : DataTypeConversion
  Data Type Conversion3 : DataTypeConversion  OutDataTypeStr=boolean
  Data Type Conversion4 : DataTypeConversion  OutDataTypeStr=int8
  Data Type Conversion5 : DataTypeConversion
  Detect Change : simulink/Logic and Bit Operations/Detect Change  vinit=0  InputProcessing=Inherited  OutDataTypeStr=boolean
  EnableInverterOvrrideSW : Constant  Value=0
  EnableInverterOvrrideVal : Constant  Value=0
  HVCAN_State : Constant
  INVpower_OvrrdSwtch : Constant  Value=0
  INVpower_OvrrdValue : Constant
  "MCU_Manager " : Stateflow chart  RequirementInfo={} %GIDa_0a8568ff_cac9_407a_8ad1_37fb58dfb6cf  TreatAsAtomicUnit=on
  Memory : Memory
  Memory1 : Memory
  ReqStateOVrRDSwitch : Constant  Value=0
  RequestedStateOvrRdValue : Constant
  ShutdownCurrent : Constant  Value=0.5
  Switch : Switch  Criteria=u2 > Threshold
  Switch1 : Switch  Criteria=u2 > Threshold
  Switch5 : Switch  Criteria=u2 > Threshold
  MCU_Status : Outport
  MCU_CAN : Outport  Port=2
  MCU_Relay : Outport  Port=3
  wires:
  Memory1/1 -> Data Type Conversion5/1
  Memory/1 -> Data Type Conversion1/1
  "MCU_Manager "/2(INVCON_Power) -> Switch5/3  "INVCON_Power"
  INVpower_OvrrdValue/1 -> Switch5/1
  INVpower_OvrrdSwtch/1 -> Switch5/2
  Data Type Conversion5/1 -> "MCU_Manager "/3(HV_State)
  Bus Selector/3 -> Memory1/1  "<HV_State>"
  Bus Selector3/1 -> Detect Change/1  "<MessageCounter_200>"
  Data Type Conversion4/1 -> "MCU_Manager "/6(KeyPos)
  Bus Selector3/2 -> Data Type Conversion4/1  "<SysPwrMd>"
  Bus Selector3/3 -> "MCU_Manager "/7(LinkVoltage)  "<BMS_Spannung_ZwKr>"
  EnableInverterOvrrideSW/1 -> Switch1/2
  Bus Selector1/1 -> Switch1/3  "<EnableInverter>"
  Switch1/1 -> Memory/1
  Control/1 -> Bus Selector1/1
  RequestedStateOvrRdValue/1 -> Switch/1
  ReqStateOVrRDSwitch/1 -> Switch/2
  "MCU_Manager "/3(RequestedStateINV) -> Switch/3  "VCU_RequestedStateINVOut"
  Switch/1 -> Bus Creator3/1  "VCU_RequestedStateINV"
  "MCU_Manager "/4(CAN_Activation) -> Bus Creator3/2  "VCU_flgInvrCanActvnCmd"
  Detect Change/1 -> "MCU_Manager "/5(INVCON_Power_Feedback)  "INVCON_Power_Feedback"
  Data Type Conversion3/1 -> "MCU_Manager "/2(ReadyToCharge)
  Bus Selector/2 -> Data Type Conversion3/1  "<ReadyToCharge>"
  Data Type Conversion2/1 -> "MCU_Manager "/4(HVCAN_State)  "HVCAN_State"
  Bus Creator3/1 -> MCU_CAN/1
  Sensors/1 -> Bus Selector3/1  "Sensors"
  EnableInverterOvrrideVal/1 -> Switch1/1
  HV_Bus_Status/1 -> Bus Selector/1  "HV_Bus Status"
  Bus Selector/1 -> Data Type Conversion/1  "<ReadyToDrive>"
  ShutdownCurrent/1 -> "MCU_Manager "/11(ShutdownCurrent)  "ShutdownCurrent"
  Bus Selector3/5 -> "MCU_Manager "/9(INV_CurrentHV)  "<INV_CurrentHV>"
  "MCU_Manager "/1(MCU_State) -> Bus Creator2/1  "MCU_State"
  Bus Creator2/1 -> MCU_Status/1
  Switch5/1 -> Bus Creator4/1  "INVCON_Power"
  Bus Creator4/1 -> MCU_Relay/1
  Data Type Conversion/1 -> "MCU_Manager "/1(ReadyToDrive)
  Data Type Conversion1/1 -> "MCU_Manager "/10(EnableInverter)
  Bus Selector3/4 -> "MCU_Manager "/8(INV_State)  "<INV_State>"
  HVCAN_State/1 -> Data Type Conversion2/1  "HVCAN_State"

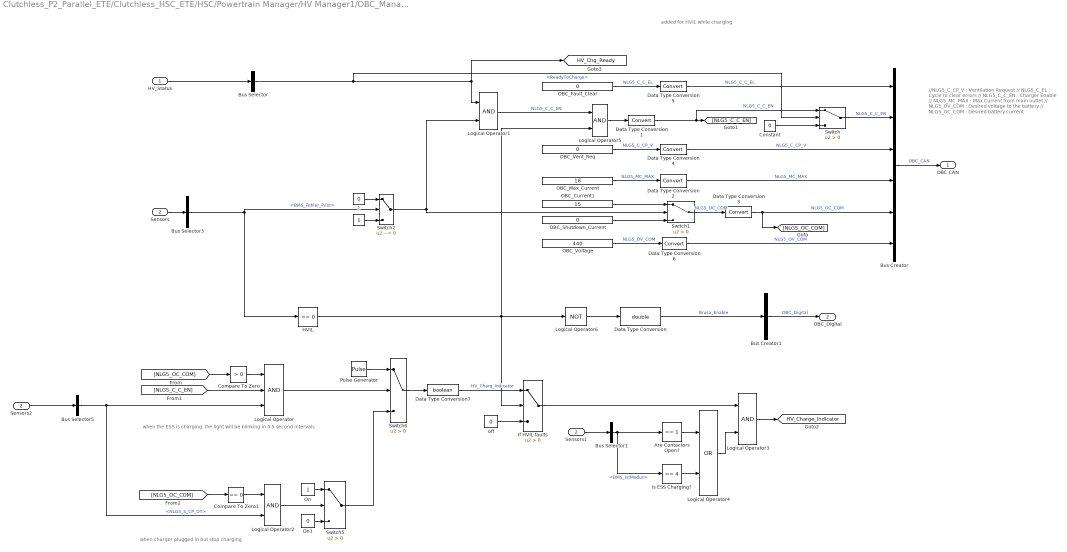
== system Clutchless_P2_Parallel_ETE/Clutchless_HSC_ETE/HSC/Powertrain Manager/HV Manager1/OBC_Manager ==
  note: when the ESS is charging, the light will be blinking in 0.5 second intervals
  note: when charger plugged in but stop charging
  note: //NLG5_C_CP_V : Ventilation Request
      | // NLG5_C_EL : Cycle to clear errors
      | // NLG5_C_C_EN : Charger Enable
      | // NLG5_MC_MAX : Max Current from main outlet
      | // NLG5_OV_COM : Desired voltage to the battery
      | // NLG5_OC_COM : Desired battery current
  note: added for HVIL
      | while charging
  HV_Status : Inport
  Sensors : Inport  Port=2
  " " : Constant
  "   1" : Constant  Value=0
  Are Contactors Open? : simulink/Logic and Bit Operations/Compare To Constant  relop===  const=1  OutDataTypeStr=boolean
  Bus Creator : BusCreator  Inputs=6
  Bus Creator1 : BusCreator  Inputs=1
  Bus Selector : BusSelector  OutputSignals=ReadyToCharge
  Bus Selector1 : BusSelector  OutputSignals=from_CAN.fromHV_CAN.from_BMSHybrid.BMS_HYB_02.BMS_IstModus
  Bus Selector3 : BusSelector  OutputSignals=from_CAN.fromHV_CAN.from_BMSHybrid.BMS_HYB_02.BMS_Fehler_Pilot
  Bus Selector5 : BusSelector  OutputSignals=from_CAN.fromHV_CAN.from_OBC.NLG5_ST.NLG5_S_CP_DT
  Compare To Zero : simulink/Logic and Bit Operations/Compare To Zero  relop=>  OutDataTypeStr=boolean
  Compare To Zero1 : simulink/Logic and Bit Operations/Compare To Zero  relop===  OutDataTypeStr=boolean
  Constant : Constant  Value=0
  Data Type Conversion : DataTypeConversion  OutDataTypeStr=double
  Data Type Conversion{1..6} (6 alike) : DataTypeConversion
  Data Type Conversion7 : DataTypeConversion  OutDataTypeStr=boolean
  HVIL : simulink/Logic and Bit Operations/Compare To Constant  relop===  const=0  OutDataTypeStr=boolean
  If HVIL faults : Switch  Criteria=u2 > Threshold
  Is ESS Charging? : simulink/Logic and Bit Operations/Compare To Constant  relop===  const=4  OutDataTypeStr=boolean
  Logical Operator : Logic  Inputs=3  AllPortsSameDT=off  OutDataTypeStr=boolean
  Logical Operator{1..3,5} (4 alike) : Logic  AllPortsSameDT=off  OutDataTypeStr=boolean
  Logical Operator4 : Logic  Operator=OR  AllPortsSameDT=off  OutDataTypeStr=boolean
  Logical Operator6 : Logic  Operator=NOT  Inputs=3  AllPortsSameDT=off  OutDataTypeStr=boolean
  OBC_Current1 : Constant  Value=15
  OBC_Fault_Clear : Constant  Value=0
  OBC_Max_Current : Constant  Value=18
  OBC_Shutdown_Current : Constant  Value=0
  OBC_Vent_Req : Constant  Value=0
  OBC_Voltage : Constant  Value=440
  On : Constant
  On1 : Constant  Value=0
  Pulse Generator : DiscretePulseGenerator  PulseType=Time based  Period=1  PulseWidth=50
  Sensors1 : InportShadow  Port=2
  Sensors2 : InportShadow  Port=2
  Switch{,1,5..6} (4 alike) : Switch  Criteria=u2 > Threshold
  Switch2 : Switch  Criteria=u2 ~= 0
  off : Constant  Value=0
  OBC CAN : Outport
  OBC_Digital : Outport  Port=2
  tag scope: HV_Charge_Indicator=global, HV_Chg_Ready=global
  wires:
  Sensors2/1 -> Bus Selector5/1
  Switch/1 -> Bus Creator/2  "NLG5_C_C_EN"
  Constant/1 -> Switch/3
  Logical Operator6/1 -> Data Type Conversion/1
  Logical Operator5/1 -> Data Type Conversion1/1
  Logical Operator4/1 -> Logical Operator3/2
  Is ESS Charging?/1 -> Logical Operator4/2
  Bus Selector1/1 -> Are Contactors Open?/1, Is ESS Charging?/1  "<BMS_IstModus>"
  Are Contactors Open?/1 -> Logical Operator4/1
  Sensors1/1 -> Bus Selector1/1
  Logical Operator3/1 -> [HV_Charge_Indicator]
  off/1 -> If HVIL faults/3
  If HVIL faults/1 -> Logical Operator3/1
  HVIL/1 -> Logical Operator5/2, If HVIL faults/2, Logical Operator6/1
  "   1"/1 -> Switch2/1
  " "/1 -> Switch2/3
  Bus Creator1/1 -> OBC_Digital/1  "OBC_Digital"
  Data Type Conversion/1 -> Bus Creator1/1  "Brusa_Enable"
  Bus Selector3/1 -> Switch2/2, HVIL/1  "<BMS_Fehler_Pilot>"
  Bus Selector5/1 -> Logical Operator/3, Logical Operator2/2  "<NLG5_S_CP_DT>"
  Switch6/1 -> Data Type Conversion7/1
  Switch5/1 -> Switch6/3
  On1/1 -> Switch5/3
  On/1 -> Switch5/1
  Logical Operator2/1 -> Switch5/2
  Compare To Zero1/1 -> Logical Operator2/1
  [NLG5_OC_COM] -> Compare To Zero1/1
  Pulse Generator/1 -> Switch6/1
  Logical Operator/1 -> Switch6/2
  [NLG5_C_C_EN] -> Logical Operator/2
  Compare To Zero/1 -> Logical Operator/1
  [NLG5_OC_COM] -> Compare To Zero/1
  Sensors/1 -> Bus Selector3/1
  Bus Creator/1 -> OBC CAN/1  "OBC_CAN"
  HV_Status/1 -> Bus Selector/1
  Bus Selector/1 -> [HV_Chg_Ready], Logical Operator1/1, Switch/2  "<ReadyToCharge>"
  Switch2/1 -> Logical Operator1/2, Switch1/2
  Data Type Conversion2/1 -> Bus Creator/4  "NLG5_MC_MAX"
  Data Type Conversion5/1 -> Bus Creator/1  "NLG5_C_C_EL"
  Data Type Conversion4/1 -> Bus Creator/3  "NLG5_C_CP_V"
  Data Type Conversion6/1 -> Bus Creator/6  "NLG5_OV_COM"
  Data Type Conversion3/1 -> [NLG5_OC_COM], Bus Creator/5  "NLG5_OC_COM"
  OBC_Current1/1 -> Switch1/1
  OBC_Shutdown_Current/1 -> Switch1/3
  Data Type Conversion1/1 -> [NLG5_C_C_EN], Switch/1  "NLG5_C_C_EN"
  Logical Operator1/1 -> Logical Operator5/1  "NLG5_C_C_EN"
  Switch1/1 -> Data Type Conversion3/1  "NLG5_OC_COM"
  OBC_Vent_Req/1 -> Data Type Conversion4/1  "NLG5_C_CP_V"
  OBC_Fault_Clear/1 -> Data Type Conversion5/1  "NLG5_C_C_EL"
  OBC_Max_Current/1 -> Data Type Conversion2/1  "NLG5_MC_MAX"
  OBC_Voltage/1 -> Data Type Conversion6/1  "NLG5_OV_COM"
  Data Type Conversion7/1 -> If HVIL faults/1  "HV_Charg_Indicator"

== system Clutchless_P2_Parallel_ETE/Clutchless_HSC_ETE/HSC/Powertrain Manager/Thermal Manager/Cooling Fan Manger ==
  Temp : Inport
  Bus Selector : BusSelector  OutputSignals=Temp_Signals.EngCltTmp,Temp_Signals.BMS_Temperatur,Temp_Signals.INV_ElectricMachineTemperature,Temp_Signals.INV_InverterTemperature,VehSpdAvgDrvn,Component_State.SysPwrMd
  Constant : Constant  Value=0
  ESSTargTemp : RelationalOperator  OutDataTypeStr=boolean  RndMeth=Nearest
  EnTargTemp : RelationalOperator  OutDataTypeStr=boolean  RndMeth=Nearest
  EnTargTemp1 : RelationalOperator  Operator=>  OutDataTypeStr=boolean  RndMeth=Nearest
  Fan_Disable : Constant  Value=0
  Fan_Enable : Constant
  Fan_EngTempThrshld : Constant  Value=100
  Fan_EssTempThrshld : Constant  Value=25
  Fan_MCUTempThrshld : Constant  Value=35
  Fan_MotTempThrshld : Constant  Value=35
  Fan_VehSpdThrshld : Constant  Value=10
  InvTargTemp : RelationalOperator  OutDataTypeStr=boolean  RndMeth=Nearest
  InvTargTemp1 : RelationalOperator  Operator=<=  OutDataTypeStr=boolean  RndMeth=Nearest
  Logical Operator : Logic  Operator=OR  Inputs=4  AllPortsSameDT=off  OutDataTypeStr=boolean
  Logical Operator1 : Logic  AllPortsSameDT=off  OutDataTypeStr=boolean
  Logical Operator2 : Logic  AllPortsSameDT=off  OutDataTypeStr=boolean
  MorTargTemp : RelationalOperator  OutDataTypeStr=boolean  RndMeth=Nearest
  Switch : Switch  Criteria=u2 ~= 0
  Fan_control : Outport
  wires:
  Fan_VehSpdThrshld/1 -> InvTargTemp1/2
  Fan_MCUTempThrshld/1 -> InvTargTemp/2
  Fan_MotTempThrshld/1 -> MorTargTemp/2
  Fan_EssTempThrshld/1 -> ESSTargTemp/2
  Fan_EngTempThrshld/1 -> EnTargTemp/2
  InvTargTemp1/1 -> Logical Operator1/2
  Bus Selector/5 -> InvTargTemp1/1  "<VehSpdAvgDrvn>"
  Logical Operator/1 -> Logical Operator1/1
  InvTargTemp/1 -> Logical Operator/4
  MorTargTemp/1 -> Logical Operator/3
  ESSTargTemp/1 -> Logical Operator/2
  EnTargTemp/1 -> Logical Operator/1
  Bus Selector/4 -> InvTargTemp/1  "<INV_InverterTemperature>"
  Bus Selector/3 -> MorTargTemp/1  "<INV_ElectricMachineTemperature>"
  Bus Selector/2 -> ESSTargTemp/1  "<BMS_Temperatur>"
  Bus Selector/1 -> EnTargTemp/1  "<EngCltTmp>"
  Fan_Enable/1 -> Switch/1
  Fan_Disable/1 -> Switch/3
  Switch/1 -> Fan_control/1
  Temp/1 -> Bus Selector/1
  Logical Operator2/1 -> Switch/2
  Logical Operator1/1 -> Logical Operator2/1
  EnTargTemp1/1 -> Logical Operator2/2
  Bus Selector/6 -> EnTargTemp1/1  "<SysPwrMd>"
  Constant/1 -> EnTargTemp1/2

== system Clutchless_P2_Parallel_ETE/Clutchless_HSC_ETE/HSC/Powertrain Manager/Thermal Manager/ESS Pump Manger ==
  note: If ESS temp>35°，enable pump100 and cooling fan and 2-way valve then enable AC-compressor
      |
      | If 35°>ESStemp≥23°，enable pump100 and cooling fan
      |
      | If 23°>ESS temp disable
      |
      | If 15°>ESS temp, enable heat coolant
  ESS_temp : Inport
  Bus Creator : BusCreator  Inputs=4
  Bus Selector : BusSelector  OutputSignals=Temp_Signals.BMS_Temperatur,Component_State.SysPwrMd
  Chart1 : Stateflow chart  TreatAsAtomicUnit=on
  ESS_Comp_TempThrs : Constant  Value=35
  ESS_Temp_State_1_Thrs : Constant  Value=15
  ESS_Temp_State_2_Thrs : Constant  Value=25
  ESS_Temp_State_3_Thrs : Constant  Value=35
  ESS_Thermal_Control : Outport
  wires:
  Bus Creator/1 -> ESS_Thermal_Control/1
  ESS_Comp_TempThrs/1 -> Chart1/5(ESS_Comp_TempThrs)
  ESS_Temp_State_3_Thrs/1 -> Chart1/4(ESS_Temp_State_3_Thrs)
  ESS_Temp_State_2_Thrs/1 -> Chart1/3(ESS_Temp_State_2_Thrs)
  ESS_Temp_State_1_Thrs/1 -> Chart1/2(ESS_Temp_State_1_Thrs)
  Chart1/3(ESS_val) -> Bus Creator/3  "ESS_val"
  Chart1/2(ESS_pump_control) -> Bus Creator/2  "ESS_pump_control"
  Chart1/1(ESS_comp) -> Bus Creator/1  "ESS_comp"
  Bus Selector/1 -> Chart1/1(ESS_temp), Chart1/6(ESS_CltTemp)  "<BMS_Temperatur>"
  ESS_temp/1 -> Bus Selector/1
  Chart1/4(ESS_comp_Enable) -> Bus Creator/4  "ESS_Comp_Enable"
  Bus Selector/2 -> Chart1/7(SysPowMod)  "<SysPwrMd>"

== system Clutchless_P2_Parallel_ETE/Clutchless_HSC_ETE/HSC/Powertrain Manager/Thermal Manager/MotInv Pump Manger ==
  MotInv_temp : Inport
  Bus Selector : BusSelector  OutputSignals=Temp_Signals.INV_ElectricMachineTemperature,Temp_Signals.INV_InverterTemperature,Component_State.SysPwrMd
  MCUPump_Manager : Stateflow chart  TreatAsAtomicUnit=on
  MCU_Temp_State_1_Thrs : Constant  Value=30
  MCU_Temp_State_2_Thrs : Constant  Value=50
  Mot_Temp_State_1_Thrs : Constant  Value=30
  Mot_Temp_State_2_Thrs1 : Constant  Value=45
  MotInvpump_control : Outport
  wires:
  MCU_Temp_State_2_Thrs/1 -> MCUPump_Manager/6(Mot_Temp_State_2_Thrs)
  Mot_Temp_State_2_Thrs1/1 -> MCUPump_Manager/5(MCU_Temp_State_2_Thrs)
  Mot_Temp_State_1_Thrs/1 -> MCUPump_Manager/3(MCU_Temp_State_1_Thrs)
  MCU_Temp_State_1_Thrs/1 -> MCUPump_Manager/4(Mot_Temp_State_1_Thrs)
  Bus Selector/2 -> MCUPump_Manager/2(MCU_temp)  "<INV_InverterTemperature>"
  Bus Selector/1 -> MCUPump_Manager/1(Motor_temp)  "<INV_ElectricMachineTemperature>"
  MotInv_temp/1 -> Bus Selector/1
  Bus Selector/3 -> MCUPump_Manager/7(SysPowMod)  "<SysPwrMd>"
  MCUPump_Manager/1(MotInvpump_control) -> MotInvpump_control/1

== system Clutchless_P2_Parallel_ETE/Clutchless_HSC_ETE/HSC/Powertrain Manager/Torque Distribution/AxlTrq_to_EngTrq ==
  note: //From engine axle torque to engine torque//
  note: check this rate limiter
  In1 : Inport
  Compare To Constant : simulink/Logic and Bit Operations/Compare To Constant  relop===  const=0  OutDataTypeStr=boolean
  Constant1 : Constant  Value=max(gb.plant.init.ratio.map)
  Constant5 : Constant  Value=fd.plant.init.ratio
  Divide1 : Product  Inputs=*//
  Ground : Ground  Commented=on
  Rate Limiter : RateLimiter  RisingSlewLimit=1000  FallingSlewLimit=-2000
  Rate Limiter1 : RateLimiter  Commented=on  RisingSlewLimit=Engine.trq_uprate  FallingSlewLimit=Engine.trq_derate
  Ratio Filter : Subsystem
  Switch : Switch  Criteria=u2 > Threshold
  Terminator : Terminator  Commented=on
  Out1 : Outport
  wires:
  Ground/1 -> Rate Limiter1/1
  Rate Limiter1/1 -> Terminator/1
  Ratio Filter/1(Filtered_Ratio) -> Compare To Constant/1, Switch/3
  Rate Limiter/1 -> Out1/1
  Switch/1 -> Divide1/3
  Constant1/1 -> Switch/1
  Compare To Constant/1 -> Switch/2
  [TransRatio] -> Ratio Filter/1(Ratio)
  Divide1/1 -> Rate Limiter/1
  Constant5/1 -> Divide1/2
  In1/1 -> Divide1/1

== system Clutchless_P2_Parallel_ETE/Clutchless_HSC_ETE/HSC/Powertrain Manager/Torque Distribution/AxlTrq_to_MotTrq ==
  In1 : Inport
  AxlTrq_to_MtrTrq2 : Subsystem
  MotTrqLimit : Saturate  UpperLimit=250  LowerLimit=-200
  Scope : Scope  NumInputPorts=4
  electric machine filter : Subsystem
  Out1 : Outport
  wires:
  MotTrqLimit/1 -> Scope/3, Out1/1, Scope/4  "MtrTrqCmd"
  electric machine filter/1(filtered) -> MotTrqLimit/1, Scope/2  "MtrTrqCmd"
  AxlTrq_to_MtrTrq2/1(MtrTrqCmd) -> electric machine filter/1(trq), Scope/1  "MtrTrqCmd"
  In1/1 -> AxlTrq_to_MtrTrq2/1(In1)

== system Clutchless_P2_Parallel_ETE/Clutchless_HSC_ETE/HSC/Powertrain Manager/Torque Distribution/RegTrqLimit ==
  MotTrqCmd : Inport
  RPM : Inport  Port=2
  Compare To Constant : simulink/Logic and Bit Operations/Compare To Constant  relop=<=  const=0  OutDataTypeStr=boolean
  Divide : Product  Inputs=**
  Regen Trq Derating2 : Lookup_n-D  NumberOfTableDimensions=1  BreakpointsForDimension1=[0 200 600 800 1000 1200 12000]  Table=[0 0.05 0.5 0.8 0.95 1 1]  ExtrapMethod=Clip  UseLastTableValue=on  InternalRulePriority=Speed  RndMeth=Simplest  InputSameDT=on
  Regen Trq Derating3 : Lookup_n-D  Commented=on  NumberOfTableDimensions=1  BreakpointsForDimension1=[0 400 800 1200 1600 2000 2400 2800]  Table=[0 0 0.2 0.5 0.8 1 1 1]  ExtrapMethod=Clip  UseLastTableValue=on  InternalRulePriority=Speed  RndMeth=Simplest  InputSameDT=on
  Regen Trq Derating4 : Lookup_n-D  Commented=on  NumberOfTableDimensions=1  BreakpointsForDimension1=[0 200 600 800 1000 1200 12000]  Table=[0 0.05 0.2 0.5 0.8 1 1]  ExtrapMethod=Clip  UseLastTableValue=on  InternalRulePriority=Speed  RndMeth=Simplest  InputSameDT=on
  Saturation : Saturate  UpperLimit=250  LowerLimit=-45
  Switch2 : Switch  Criteria=u2 > Threshold
  rpm2rads : Gain  Gain=9.549
  Out1 : Outport
  wires:
  Regen Trq Derating2/1 -> Divide/1
  rpm2rads/1 -> Regen Trq Derating2/1
  Divide/1 -> Switch2/1
  Compare To Constant/1 -> Switch2/2
  RPM/1 -> rpm2rads/1
  Switch2/1 -> Saturation/1
  MotTrqCmd/1 -> Compare To Constant/1, Divide/2, Switch2/3
  Saturation/1 -> Out1/1

== system Clutchless_P2_Parallel_ETE/Clutchless_HSC_ETE/HSC/Powertrain Manager/Torque Distribution/Select_APP ==
  APP_Select : Constant  Value=0
  Data Type Conversion10 : DataTypeConversion  OutDataTypeStr=boolean
  Switch1 : Switch  Criteria=u2 > Threshold
  EngAppReq : Outport
  wires:
  [EngAppReq] -> Switch1/3
  [AccPos_Perc] -> Switch1/1
  Data Type Conversion10/1 -> Switch1/2
  APP_Select/1 -> Data Type Conversion10/1
  Switch1/1 -> EngAppReq/1  "EngAppReq"

== system Clutchless_P2_Parallel_ETE/Clutchless_HSC_ETE/HSC/Powertrain Manager/Torque Distribution/Sport Mode Enable ==
  In1 : Inport
  Bus Selector5 : BusSelector  OutputSignals=from_Analog.Sport_Mode_SW
  Compare To Constant : simulink/Logic and Bit Operations/Compare To Constant  relop===  const=2  OutDataTypeStr=boolean
  Sports Mode Logic : Stateflow chart  TreatAsAtomicUnit=on
  Out1 : Outport
  wires:
  In1/1 -> Bus Selector5/1
  Bus Selector5/1 -> Sports Mode Logic/1(Voltage_Input)  "<Sport_Mode_SW>"
  Sports Mode Logic/1(Driver_Mode) -> Compare To Constant/1
  Compare To Constant/1 -> Out1/1

== system Clutchless_P2_Parallel_ETE/Clutchless_HSC_ETE/HSC/Powertrain Manager/Torque Distribution/Subsystem1 ==
  SoC : Inport
  CS_On : Inport  Port=2
  Constant : Constant
  Sample and Hold1 : dspsigops/Sample and Hold  trig=Rising edge  initCond=0  latchinput=off
  Switch : Switch  Criteria=u2 > Threshold
  Faked_SoC : Outport
  wires:
  SoC/1 -> Sample and Hold1/1
  CS_On/1 -> Switch/2, Sample and Hold1/Trigger
  Switch/1 -> Faked_SoC/1
  Sample and Hold1/1 -> Switch/1
  Constant/1 -> Switch/3
